simulink model "UbicacionDePolos_2015"  (R2015a)
settings: Solver=ode45  SolverMode=SingleTasking  StartTime=0.0  StopTime=10.0  RelTol=1e-3
settings Model: CovMetricSettings=dwe  CovHtmlReporting=off  covSaveCumulativeToWorkspaceVar=off  CovSaveSingleToWorkspaceVar=off  CovExternalEMLEnable=on  Creator=Jesus  LastModifiedBy=Jesus
settings DataIOCC: LimitDataPoints=off  SaveFormat=Dataset
settings DebuggingCC: SFUnexpectedBacktrackingDiag=error  SFNoUnconditionalDefaultTransitionDiag=error
settings HardwareCC: ProdBitPerPointer=64  ProdLargestAtomicFloat=Float  ProdIntDivRoundTo=Zero  ProdEndianess=LittleEndian  ProdHWDeviceType=Specified
settings ModelReferenceCC: PropagateSignalLabelsOutOfModel=on
settings GRTTargetCC: TargetLangStandard=C99 (ISO)  GeneratePreprocessorConditionals=Use local settings

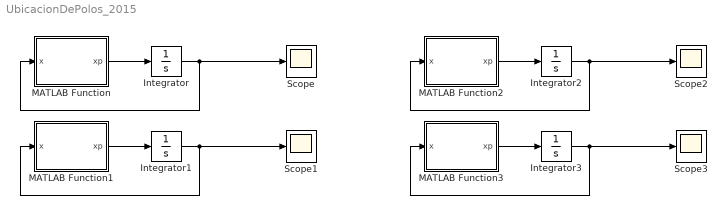
== system UbicacionDePolos_2015 ==
  Integrator{,1..3} (4 alike) : Integrator  InitialCondition=[0 0]
  MATLAB Function : MATLAB Function  TreatAsAtomicUnit=on
      settings: PermitHierarchicalResolution=ParametersOnly
  MATLAB Function1 : MATLAB Function  TreatAsAtomicUnit=on
      settings: PermitHierarchicalResolution=ParametersOnly
  MATLAB Function2 : MATLAB Function  TreatAsAtomicUnit=on
      settings: PermitHierarchicalResolution=ParametersOnly
  MATLAB Function3 : MATLAB Function  TreatAsAtomicUnit=on
      settings: PermitHierarchicalResolution=ParametersOnly
  Scope{,1..3} (4 alike) : Scope
      Scope settings: TimeRange=auto  MaxDataPoints=5000  SaveToWorkspace=off  SaveName=ScopeData  YMin=-3680031784482884.00000  YMax=33120286060345964.00000  SampleTime=-1
      Scope1 settings: TimeRange=auto  MaxDataPoints=5000  SaveToWorkspace=off  YMin=-0.40251  YMax=0.84674  SampleTime=-1
      Scope2 settings: TimeRange=auto  MaxDataPoints=5000  SaveToWorkspace=off  SaveName=ScopeData2  YMin=-3680031784482884.00000  YMax=33120286060345964.00000  SampleTime=-1
      Scope3 settings: TimeRange=auto  MaxDataPoints=5000  SaveToWorkspace=off  SaveName=ScopeData3  YMin=-0.40251  YMax=0.84674  SampleTime=-1
  wires:
  MATLAB Function/1(xp) -> Integrator/1
  Integrator/1 -> Scope/1, MATLAB Function/1(x)
  Integrator1/1 -> MATLAB Function1/1(x), Scope1/1
  MATLAB Function1/1(xp) -> Integrator1/1
  MATLAB Function3/1(xp) -> Integrator3/1
  Integrator3/1 -> Scope3/1, MATLAB Function3/1(x)
  Integrator2/1 -> MATLAB Function2/1(x), Scope2/1
  MATLAB Function2/1(xp) -> Integrator2/1

== matlab function UbicacionDePolos_2015/MATLAB Function1 ==
  data: x input; xp output
function xp = fcn(x)
r=1;
K=[4,5.6667];
u=r-K*x;
A = [1 3;3 1];
B = [1 0]';
xp = A*x+B*u;

== matlab function UbicacionDePolos_2015/MATLAB Function ==
  data: x input; xp output
function xp = fcn(x)
u=1;
A = [1 3;3 1];
B = [1 0]';
xp = A*x+B*u;

== matlab function UbicacionDePolos_2015/MATLAB Function2 ==
  data: x input; xp output
function xp = fcn(x)
u=1;
A = [1 3;3 1];
B = [1 0]';
xp = A*x+B*u;

== matlab function UbicacionDePolos_2015/MATLAB Function3 ==
  data: x input; xp output
function xp = fcn(x)
r=1;
K=[3.5,4];
u=r-K*x;
A = [1 3;3 1];
B = [1 0]';
xp = A*x+B*u;
